simulink library "displays"  (Simulink 8.5)
settings: Solver=ode45  SolverMode=SingleTasking  StartTime=0.0  StopTime=10.0  RelTol=1e-3
values from neighbouring files (symbols this model uses):
  h = uimenu('Label','QUIT')    [M2Kc.M]
  h2 = uimenu(h1,'Label','Distance')    [M2Kc.M]
undefined symbols (not defined in the file or in its folder): fig, H_ang, H_mag, type
settings Model: Creator=PC  LastModifiedBy=PC

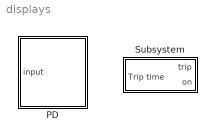
== system displays ==
  PD : Subsystem  mask(Phasor Display){Bactive=off, type1=transient, dint=0.1}
      mask prompts: Bactive "Block active"; type1 "Display type"; dint "Display intervals(sec):"
      mask help: Displays the phasor(s) dynamically on the complex plane. Its inputs are the magnitude and angle (in degrees) of each phasor. Up to six phasors can be displayed. There are two types of display: transient and steady state. In the former, the display interval must be entered, while in the latter, the block displays the value of the phasor(s) at the end of the simulation.
      mask init:
      | pd0;
      mask TypeOptions type1: transient | steady state
      mask Display: disp('Phasor\nDisplay');
  Subsystem : Subsystem

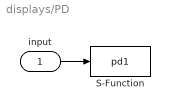
== system displays/PD ==
  input : Inport
  S-Function : S-Function  FunctionName=pd1  Parameters=Bactive,type,dint,h,h2,H_mag,H_ang,fig
  wires:
  input/1 -> S-Function/1

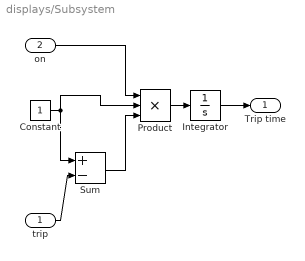
== system displays/Subsystem ==
  trip : Inport
  on : Inport  Port=2
  Constant : Constant
  Integrator : Integrator
  Product : Product  Inputs=3  SaturateOnIntegerOverflow=on  RndMeth=Zero  InputSameDT=on  OutDataTypeStr=Inherit: Same as first input
  Sum : Sum  Inputs=+-  SaturateOnIntegerOverflow=on  InputSameDT=on  OutDataTypeStr=Inherit: Same as first input
  Trip time : Outport  InitialOutput=0
  wires:
  on/1 -> Product/1
  Sum/1 -> Product/3
  Integrator/1 -> Trip time/1
  Product/1 -> Integrator/1
  Constant/1 -> Sum/1, Product/2
  trip/1 -> Sum/2
